simulink model "Exp4_19EE10011"  (R2021a)
settings: Solver=VariableStepAuto  StartTime=0.0  StopTime=3  RelTol=1e-3
libraries: spsSeriesRLCBranchLib x20, spsDiodeLib x13, spsCurrentMeasurementLib x11, spsVoltageMeasurementLib x9, spsThyristorLib x6, spsGroundLib x4, spsParallelRLCBranchLib x4, spsACVoltageSourceLib x3, spsLinearTransformerLib x3, spsRMSLib x2, spsMonostableLib x2, spsMosfetLib x2
settings Model: Creator=Asus  LastModifiedBy=Asus

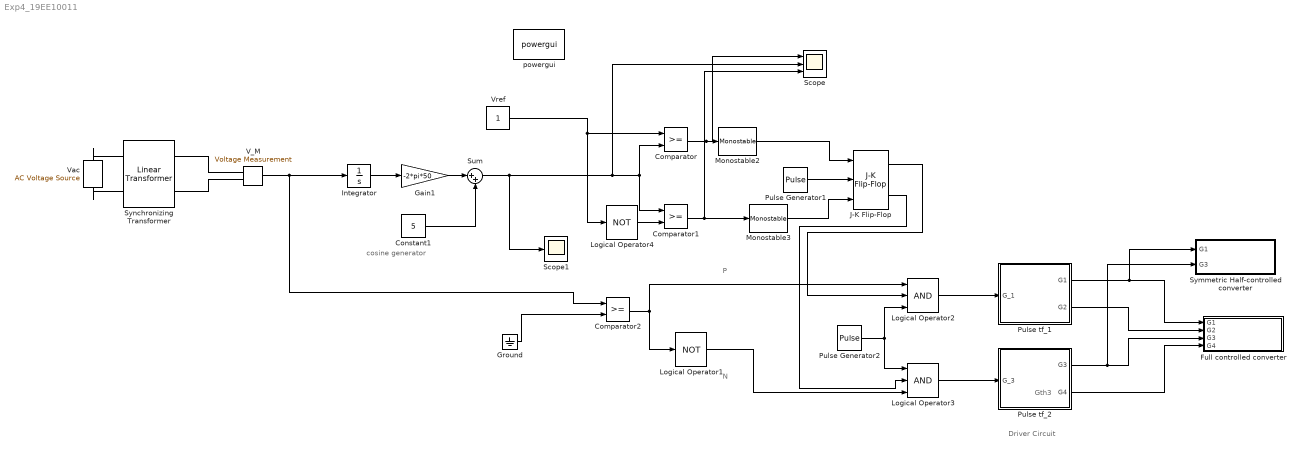
== system Exp4_19EE10011 ==
  note: Driver Circuit
  note: cosine generator
  note: P
  note: N
  note: Gth3
  Comparator : RelationalOperator  OutDataTypeStr=boolean  RndMeth=Nearest
  Comparator1 : RelationalOperator  OutDataTypeStr=boolean  RndMeth=Nearest
  Comparator2 : RelationalOperator  OutDataTypeStr=boolean  RndMeth=Nearest
  Constant1 : Constant  Value=5
  Full controlled converter : Subsystem
  Gain1 : Gain  Gain=-2*pi*50
  Ground : Ground
  Integrator : Integrator
  J-K Flip-Flop : simulink_extras/Flip Flops/J-K Flip-Flop  initial_condition=0
  Logical Operator1 : Logic  Operator=NOT  Inputs=inv  IconShape=distinctive  AllPortsSameDT=off  OutDataTypeStr=boolean
  Logical Operator2 : Logic  Inputs=3  IconShape=distinctive  AllPortsSameDT=off  OutDataTypeStr=boolean
  Logical Operator3 : Logic  Inputs=3  IconShape=distinctive  AllPortsSameDT=off  OutDataTypeStr=boolean
  Logical Operator4 : Logic  Operator=NOT  Inputs=inv  IconShape=distinctive  AllPortsSameDT=off  OutDataTypeStr=boolean
  Monostable2 : spsMonostableLib/Monostable  EdgeDetect=Rising  PulseDuration=10e-6  ic=0  Ts=0
      settings: SourceProductBaseCode=PS
  Monostable3 : spsMonostableLib/Monostable  EdgeDetect=Rising  PulseDuration=10e-6  ic=0  Ts=0
      settings: SourceProductBaseCode=PS
  Pulse Generator1 : DiscretePulseGenerator  PulseType=Time based  Period=2e-6  PulseWidth=50
  Pulse Generator2 : DiscretePulseGenerator  PulseType=Time based  Period=40e-6  PulseWidth=50
  Pulse tf_1 : Subsystem
  Pulse tf_2 : Subsystem
  Scope : Scope  NumInputPorts=3
  Scope1 : Scope
  Sum : Sum  Inputs=|++
  Symmetric Half-controlled converter : Subsystem
  Synchronizing Transformer : spsLinearTransformerLib/Linear Transformer  UNITS=SI  NominalPower=[ 4 50 ]  winding1="[230  6.90 7.1e-3]"  winding2=[3.605 0.0017 2.1e-6]  ThreeWindings=off  winding3=[3.15e+05 0.7938 0.084225]  RmLm=[600 1.145]  Measurements=None  DataType=on
  V_M : spsVoltageMeasurementLib/Voltage Measurement  PhasorSimulation=off  OutputType=Complex  PSBequivalent=0
  Vac : spsACVoltageSourceLib/AC Voltage Source  Amplitude=230  Phase=0  Frequency=50  SampleTime=0  Measurements=None  BusType=swing  Pref=10e3  Qref=0  Qmin=-inf  Qmax=+inf
  Vref : Constant
  powergui : spspowerguiLib/powergui  Priority=1  SimulationMode=Discrete  SampleTime=1e-6  frequency=60  Iterations=50  frequencyindice=50  Pbase=100e6  ErrMax=1e-4  UnitsV=kV  UnitsW=MW  buscounter=0  FunctionMessages=off  echomessages=off  EnableUseOfTLC=off  CurrentSourceSwitches=off  DisableSnubberDevices=off  DisableRonSwitches=off  DisableVfSwitches=off  DisplayEquations=off  AutomaticDiscreteSolvers=off  SolverType=Tustin/Backward Euler (TBE)  Interpol=off  ExternalGateDelay=off  methode=off  Ts=10  x0status=blocks  SPID=off  SwTol=0  HookPort=off  NonlinearTolerance=1e-4  nMaxIteration=100  ContinueOnMaxIteration=off  RestoreLinks=warning  ResistiveCurrentMeasurement=off  Frange=[0:2:500]  Ylog=off  Xlog=on  ShowGrid=off  save=off  variable=ZData  structure=ScopeData10  ZoomFFT=off  StartTime=0.124  cycles=2  DisplayStyle=2  fundamental=50  FreqAxis=on  MaxFrequency=5000  frequencyindicesteady=1  RmsSteady=1  display=off
  wires:
  Comparator/1 -> Scope/1, Monostable2/1
  J-K Flip-Flop/2 -> Logical Operator3/2
  Comparator1/1 -> Scope/3, Monostable3/1
  Monostable2/1 -> J-K Flip-Flop/1
  Logical Operator1/1 -> Logical Operator3/3
  Pulse Generator2/1 -> Logical Operator3/1, Logical Operator2/3
  Pulse Generator1/1 -> J-K Flip-Flop/2
  Ground/1 -> Comparator2/2
  Vref/1 -> Logical Operator4/1, Comparator/1
  J-K Flip-Flop/1 -> Logical Operator2/2
  Monostable3/1 -> J-K Flip-Flop/3
  Sum/1 -> Scope1/1, Comparator/2, Comparator1/1, Scope/2
  Comparator2/1 -> Logical Operator2/1, Logical Operator1/1
  Gain1/1 -> Sum/1
  Integrator/1 -> Gain1/1
  Constant1/1 -> Sum/2
  V_M/1 -> Integrator/1, Comparator2/1
  Logical Operator4/1 -> Comparator1/2
  Logical Operator2/1 -> Pulse tf_1/1(G_1)
  Logical Operator3/1 -> Pulse tf_2/1(G_3)
  Pulse tf_1/1(G1) -> Symmetric Half-controlled converter/1(G1), Full controlled converter/1(G1)
  Pulse tf_1/2(G2) -> Full controlled converter/2(G2)
  Pulse tf_2/1(G3) -> Symmetric Half-controlled converter/2(G3), Full controlled converter/3(G3)
  Pulse tf_2/2(G4) -> Full controlled converter/4(G4)
  connections:
  V_M/LConn2 -- Synchronizing Transformer/RConn2
  Vac/RConn1 -- Synchronizing Transformer/LConn1
  Vac/LConn1 -- Synchronizing Transformer/LConn2
  Synchronizing Transformer/RConn1 -- V_M/LConn1

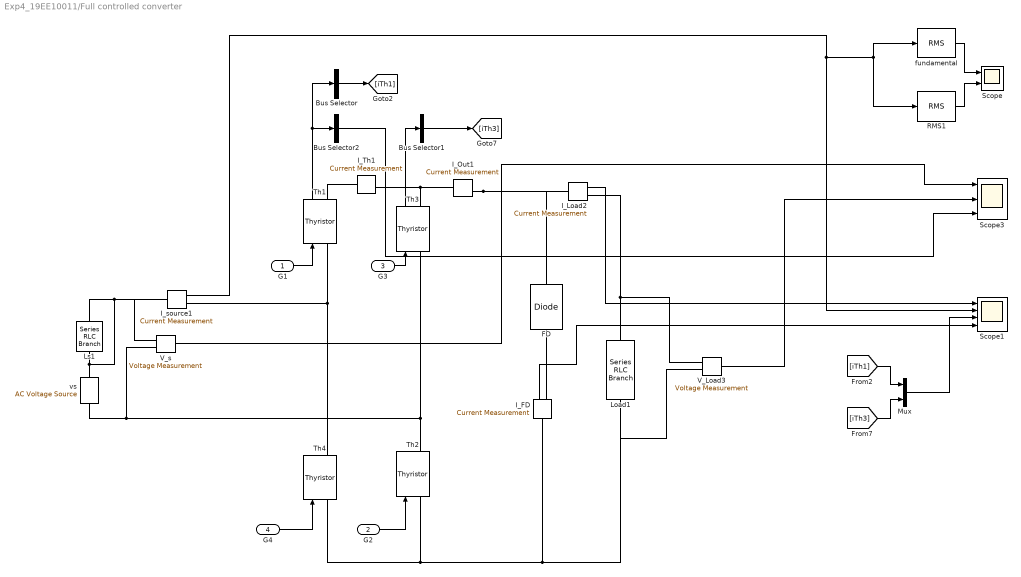
== system Exp4_19EE10011/Full controlled converter ==
  G1 : Inport
  G2 : Inport  Port=2
  G3 : Inport  Port=3
  G4 : Inport  Port=4
  Bus Selector : BusSelector  OutputSignals=Thyristor current  OutputAsBus=on
  Bus Selector1 : BusSelector  OutputSignals=Thyristor current  OutputAsBus=on
  Bus Selector2 : BusSelector  OutputSignals=Thyristor voltage  OutputAsBus=on
  FD : spsDiodeLib/Diode  Ron=0.14  Lon=0  Vf=0.6  IC=0  UseSnubber=off  Rs=500  Cs=250e-9  Measurements=off
  I_FD : spsCurrentMeasurementLib/Current Measurement  PhasorSimulation=off  OutputType=Complex  PSBequivalent=0
  I_Load2 : spsCurrentMeasurementLib/Current Measurement  PhasorSimulation=off  OutputType=Complex  PSBequivalent=0
  I_Out1 : spsCurrentMeasurementLib/Current Measurement  PhasorSimulation=off  OutputType=Complex  PSBequivalent=0
  I_Th1 : spsCurrentMeasurementLib/Current Measurement  PhasorSimulation=off  OutputType=Complex  PSBequivalent=0
  I_source1 : spsCurrentMeasurementLib/Current Measurement  PhasorSimulation=off  OutputType=Complex  PSBequivalent=0
  Load1 : spsSeriesRLCBranchLib/Series RLC Branch  LConnTagsString=__new0  RConnTagsString=__new0  BranchType=R  Resistance=22.4  Inductance=60e-3  SetiL0=off  InitialCurrent=0  Capacitance=1e-6  Setx0=off  InitialVoltage=0  Measurements=None
  Ls1 : spsSeriesRLCBranchLib/Series RLC Branch  LConnTagsString=__new0  RConnTagsString=__new0  BranchType=L  Resistance=0.01  Inductance=3.5e-3  SetiL0=off  InitialCurrent=0  Capacitance=1e-6  Setx0=off  InitialVoltage=0  Measurements=None
  Mux : Mux  Inputs=2
  RMS1 : spsRMSLib/RMS  TrueRMS=on  Freq=50  RMSInit=0  Ts=0
  Scope : Scope  NumInputPorts=2
  Scope1 : Scope  NumInputPorts=4
  Scope3 : Scope  NumInputPorts=3
  Th{1..4} (4 alike) : spsThyristorLib/Thyristor  Ron=0.05  Lon=0  Vf=1.5  IC=0  Rs=220  Cs=250e-9  Measurements=on
  V_Load3 : spsVoltageMeasurementLib/Voltage Measurement  PhasorSimulation=off  OutputType=Complex  PSBequivalent=0
  V_s : spsVoltageMeasurementLib/Voltage Measurement  PhasorSimulation=off  OutputType=Complex  PSBequivalent=0
  fundamental : spsRMSLib/RMS  TrueRMS=off  Freq=50  RMSInit=0  Ts=0
  vs : spsACVoltageSourceLib/AC Voltage Source  Amplitude=230  Phase=0  Frequency=50  SampleTime=0  Measurements=None  BusType=swing  Pref=10e3  Qref=0  Qmin=-inf  Qmax=+inf
  wires:
  Bus Selector/1 -> [iTh1]
  [iTh1] -> Mux/1
  I_FD/1 -> Scope1/4
  V_Load3/1 -> Scope3/2
  I_source1/1 -> Scope1/2, fundamental/1, RMS1/1
  G2/1 -> Th2/1
  Th1/1 -> Bus Selector/1, Bus Selector2/1
  G3/1 -> Th3/1
  G4/1 -> Th4/1
  Bus Selector2/1 -> Scope3/3
  RMS1/1 -> Scope/2
  Mux/1 -> Scope1/3
  G1/1 -> Th1/1
  I_Load2/1 -> Scope1/1
  V_s/1 -> Scope3/1
  Th3/1 -> Bus Selector1/1
  [iTh3] -> Mux/2
  Bus Selector1/1 -> [iTh3]
  fundamental/1 -> Scope/1
  connections:
  vs/LConn1 -- Th2/RConn1 -- Th3/LConn1 -- V_s/LConn2
  Th4/LConn1 -- I_FD/LConn1 -- Load1/RConn1 -- V_Load3/LConn2 -- Th2/LConn1
  I_Out1/LConn1 -- I_Th1/RConn1 -- Th3/RConn1
  V_Load3/LConn1 -- I_Load2/RConn1 -- Load1/LConn1
  Ls1/RConn1 -- Ls1/LConn1 -- V_s/LConn1 -- I_source1/LConn1 -- vs/RConn1
  I_source1/RConn1 -- Th4/RConn1 -- Th1/LConn1
  I_Out1/RConn1 -- FD/RConn1 -- I_Load2/LConn1
  Th1/RConn1 -- I_Th1/LConn1
  I_FD/RConn1 -- FD/LConn1

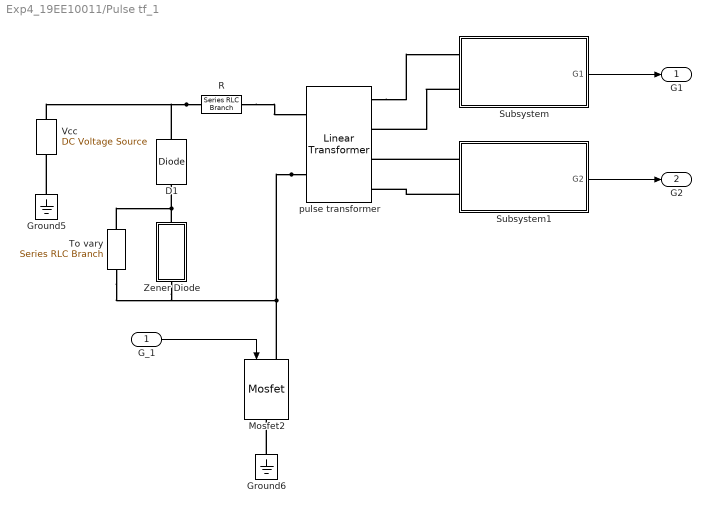
== system Exp4_19EE10011/Pulse tf_1 ==
  G_1 : Inport
  D1 : spsDiodeLib/Diode  Ron=0.001  Lon=0  Vf=0.7  IC=0  UseSnubber=off  Rs=inf  Cs=0  Measurements=off
  Ground5 : spsGroundLib/Ground  LConnTagsString=a
  Ground6 : spsGroundLib/Ground  LConnTagsString=a
  Mosfet2 : spsMosfetLib/Mosfet  Ron=0.1  Lon=0  Rd=0.01  Vfd=0  IC=0  Rs=1e5  Cs=inf  Measurements=off
  R : spsSeriesRLCBranchLib/Series RLC Branch  LConnTagsString=__new0  RConnTagsString=__new0  BranchType=R  Resistance=10  Inductance=60e-3  SetiL0=off  InitialCurrent=0  Capacitance=1e-6  Setx0=off  InitialVoltage=0  Measurements=None
  Subsystem : Subsystem
  Subsystem1 : Subsystem
  To vary : spsSeriesRLCBranchLib/Series RLC Branch  LConnTagsString=__new0  RConnTagsString=__new0  BranchType=R  Resistance=1e6  Inductance=60e-3  SetiL0=off  InitialCurrent=0  Capacitance=1e-6  Setx0=off  InitialVoltage=0  Measurements=None
  Vcc : spsDCVoltageSourceLib/DC Voltage Source  Amplitude=20  Measurements=None
  Zener Diode : Subsystem  mask(Zener Diode){Vz=30, Rzt=10, Rzk=400, Izm=10, Vf=0.7, Ron=1e-3}
      mask prompts: Vz "Zener Voltage Vz (V)"; Rzt "Dynamic Impedance Zzt (ohms)"; Rzk "Knee Impedance Zzk (ohms)"; Izm "Maximum Continuous Current Izm (A)"; Vf "Forward Voltage Drop Vf (V)"; Ron "On Resistance Ron (ohms)"
      mask help:
      | Implements a zener diode block.
      | Use values from standard datasheets to populate block dialog
  pulse transformer : spsLinearTransformerLib/Linear Transformer  UNITS=SI  NominalPower=[0.5 50e3 ]  winding1=[5 0.8 20e-6]  winding2=[5 0.8 20e-6]  ThreeWindings=on  winding3=[5 0.8 20e-6]  RmLm=[400 1.5e-3]  Measurements=None  DataType=on
  G1 : Outport
  G2 : Outport  Port=2
  wires:
  G_1/1 -> Mosfet2/1
  Subsystem1/1(G2) -> G2/1
  Subsystem/1(G1) -> G1/1
  connections:
  pulse transformer/LConn2 -- Mosfet2/LConn1 -- To vary/LConn1 -- Zener Diode/LConn1
  Ground6/LConn1 -- Mosfet2/RConn1
  Ground5/LConn1 -- Vcc/LConn1
  R/LConn1 -- pulse transformer/LConn1
  Zener Diode/RConn1 -- To vary/RConn1 -- D1/LConn1
  pulse transformer/RConn1 -- Subsystem/LConn1
  Subsystem/LConn2 -- pulse transformer/RConn2
  Subsystem1/LConn1 -- pulse transformer/RConn3
  Subsystem1/LConn2 -- pulse transformer/RConn4
  R/RConn1 -- D1/RConn1 -- Vcc/RConn1

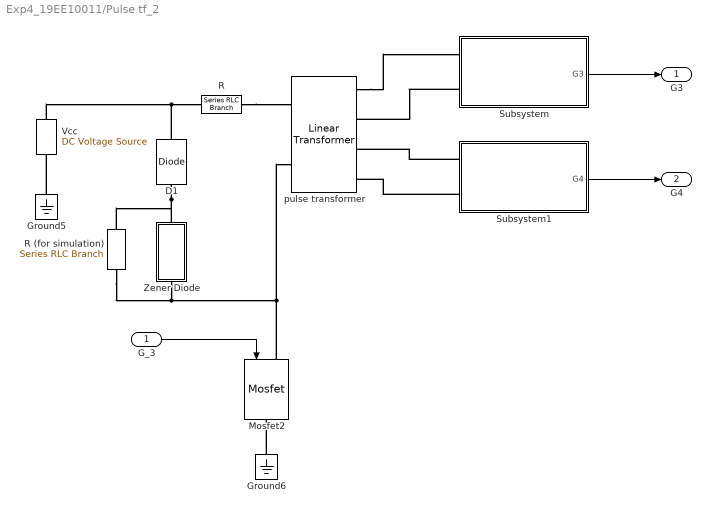
== system Exp4_19EE10011/Pulse tf_2 ==
  G_3 : Inport
  D1 : spsDiodeLib/Diode  Ron=0.001  Lon=0  Vf=0.7  IC=0  UseSnubber=off  Rs=inf  Cs=0  Measurements=off
  Ground5 : spsGroundLib/Ground  LConnTagsString=a
  Ground6 : spsGroundLib/Ground  LConnTagsString=a
  Mosfet2 : spsMosfetLib/Mosfet  Ron=0.1  Lon=0  Rd=0.01  Vfd=0  IC=0  Rs=1e5  Cs=inf  Measurements=off
  R : spsSeriesRLCBranchLib/Series RLC Branch  LConnTagsString=__new0  RConnTagsString=__new0  BranchType=R  Resistance=10  Inductance=60e-3  SetiL0=off  InitialCurrent=0  Capacitance=1e-6  Setx0=off  InitialVoltage=0  Measurements=None
  R (for simulation) : spsSeriesRLCBranchLib/Series RLC Branch  LConnTagsString=__new0  RConnTagsString=__new0  BranchType=R  Resistance=1e6  Inductance=60e-3  SetiL0=off  InitialCurrent=0  Capacitance=1e-6  Setx0=off  InitialVoltage=0  Measurements=None
  Subsystem : Subsystem
  Subsystem1 : Subsystem
  Vcc : spsDCVoltageSourceLib/DC Voltage Source  Amplitude=20  Measurements=None
  Zener Diode : Subsystem  mask(Zener Diode){Vz=30, Rzt=10, Rzk=400, Izm=10, Vf=0.7, Ron=1e-3}
      mask prompts: Vz "Zener Voltage Vz (V)"; Rzt "Dynamic Impedance Zzt (ohms)"; Rzk "Knee Impedance Zzk (ohms)"; Izm "Maximum Continuous Current Izm (A)"; Vf "Forward Voltage Drop Vf (V)"; Ron "On Resistance Ron (ohms)"
      mask help:
      | Implements a zener diode block.
      | Use values from standard datasheets to populate block dialog
  pulse transformer : spsLinearTransformerLib/Linear Transformer  UNITS=SI  NominalPower=[0.5 50e3 ]  winding1=[5 0.8 20e-6]  winding2=[5 0.8 20e-6]  ThreeWindings=on  winding3=[5 0.8 20e-6]  RmLm=[400 1.5e-3]  Measurements=None  DataType=on
  G3 : Outport
  G4 : Outport  Port=2
  wires:
  Subsystem/1(G3) -> G3/1
  Subsystem1/1(G4) -> G4/1
  G_3/1 -> Mosfet2/1
  connections:
  Vcc/RConn1 -- D1/RConn1 -- R/RConn1
  Subsystem1/LConn2 -- pulse transformer/RConn4
  Subsystem1/LConn1 -- pulse transformer/RConn3
  Subsystem/LConn2 -- pulse transformer/RConn2
  pulse transformer/RConn1 -- Subsystem/LConn1
  D1/LConn1 -- R (for simulation)/RConn1 -- Zener Diode/RConn1
  R/LConn1 -- pulse transformer/LConn1
  Ground5/LConn1 -- Vcc/LConn1
  Ground6/LConn1 -- Mosfet2/RConn1
  Zener Diode/LConn1 -- R (for simulation)/LConn1 -- Mosfet2/LConn1 -- pulse transformer/LConn2

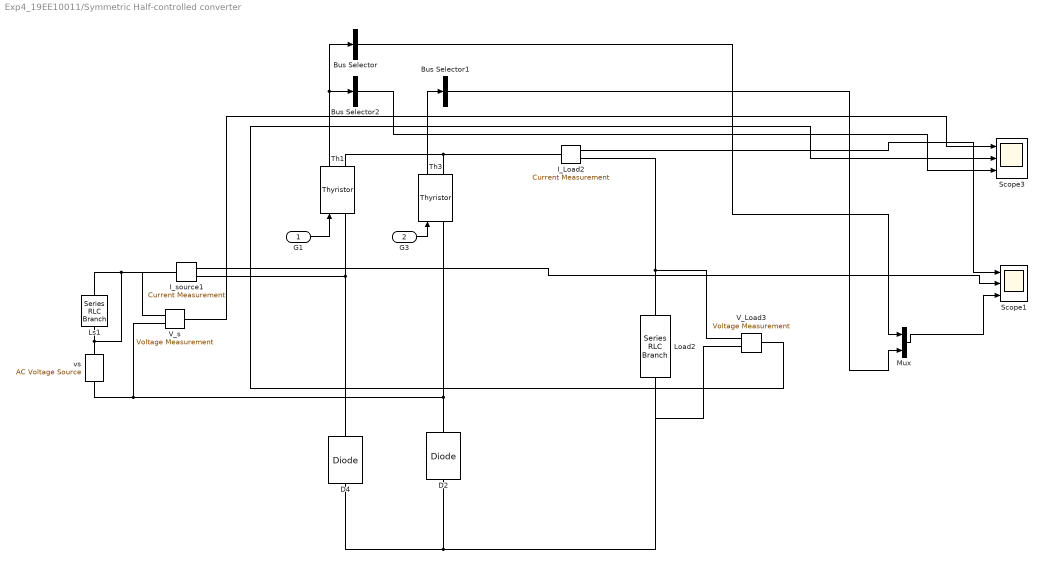
== system Exp4_19EE10011/Symmetric Half-controlled converter ==
  G1 : Inport
  G3 : Inport  Port=2
  Bus Selector : BusSelector  OutputSignals=Thyristor current  OutputAsBus=on
  Bus Selector1 : BusSelector  OutputSignals=Thyristor current  OutputAsBus=on
  Bus Selector2 : BusSelector  OutputSignals=Thyristor voltage  OutputAsBus=on
  D2 : spsDiodeLib/Diode  Ron=0.2  Lon=0  Vf=0.8  IC=0  UseSnubber=off  Rs=220  Cs=250e-9  Measurements=off
  D4 : spsDiodeLib/Diode  Ron=0.2  Lon=0  Vf=0.8  IC=0  UseSnubber=off  Rs=220  Cs=250e-9  Measurements=off
  I_Load2 : spsCurrentMeasurementLib/Current Measurement  PhasorSimulation=off  OutputType=Complex  PSBequivalent=0
  I_source1 : spsCurrentMeasurementLib/Current Measurement  PhasorSimulation=off  OutputType=Complex  PSBequivalent=0
  Load2 : spsSeriesRLCBranchLib/Series RLC Branch  LConnTagsString=__new0  RConnTagsString=__new0  BranchType=RL  Resistance=50  Inductance=60e-3  SetiL0=off  InitialCurrent=0  Capacitance=1e-6  Setx0=off  InitialVoltage=0  Measurements=None
  Ls1 : spsSeriesRLCBranchLib/Series RLC Branch  LConnTagsString=__new0  RConnTagsString=__new0  BranchType=L  Resistance=0.01  Inductance=3.5e-3  SetiL0=off  InitialCurrent=0  Capacitance=1e-6  Setx0=off  InitialVoltage=0  Measurements=None
  Mux : Mux  Inputs=2
  Scope1 : Scope  NumInputPorts=3
  Scope3 : Scope  NumInputPorts=3
  Th1 : spsThyristorLib/Thyristor  Ron=0.05  Lon=0  Vf=1.5  IC=0  Rs=220  Cs=250e-9  Measurements=on
  Th3 : spsThyristorLib/Thyristor  Ron=0.05  Lon=0  Vf=1.5  IC=0  Rs=220  Cs=250e-9  Measurements=on
  V_Load3 : spsVoltageMeasurementLib/Voltage Measurement  PhasorSimulation=off  OutputType=Complex  PSBequivalent=0
  V_s : spsVoltageMeasurementLib/Voltage Measurement  PhasorSimulation=off  OutputType=Complex  PSBequivalent=0
  vs : spsACVoltageSourceLib/AC Voltage Source  Amplitude=230  Phase=0  Frequency=50  SampleTime=0  Measurements=None  BusType=swing  Pref=10e3  Qref=0  Qmin=-inf  Qmax=+inf
  wires:
  G1/1 -> Th1/1
  Bus Selector2/1 -> Scope3/3
  Th3/1 -> Bus Selector1/1
  V_s/1 -> Scope3/1
  G3/1 -> Th3/1
  V_Load3/1 -> Scope3/2
  I_Load2/1 -> Scope1/1
  I_source1/1 -> Scope1/2
  Bus Selector/1 -> Mux/1
  Th1/1 -> Bus Selector/1, Bus Selector2/1
  Mux/1 -> Scope1/3
  Bus Selector1/1 -> Mux/2
  connections:
  D4/LConn1 -- D2/LConn1 -- V_Load3/LConn2 -- Load2/RConn1
  Ls1/RConn1 -- vs/RConn1 -- Ls1/LConn1 -- V_s/LConn1 -- I_source1/LConn1
  I_source1/RConn1 -- Th1/LConn1 -- D4/RConn1
  vs/LConn1 -- V_s/LConn2 -- Th3/LConn1 -- D2/RConn1
  I_Load2/LConn1 -- Th1/RConn1 -- Th3/RConn1
  Load2/LConn1 -- I_Load2/RConn1 -- V_Load3/LConn1

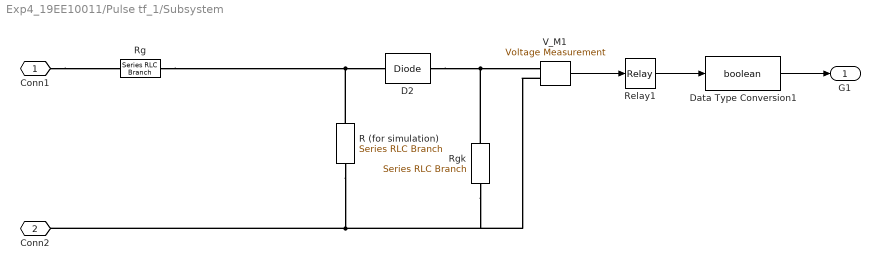
== system Exp4_19EE10011/Pulse tf_1/Subsystem ==
  D2 : spsDiodeLib/Diode  Ron=0.001  Lon=0  Vf=0.7  IC=0  UseSnubber=off  Rs=inf  Cs=0  Measurements=off
  Data Type Conversion1 : DataTypeConversion  OutDataTypeStr=boolean
  R (for simulation) : spsSeriesRLCBranchLib/Series RLC Branch  LConnTagsString=__new0  RConnTagsString=__new0  BranchType=R  Resistance=100000  Inductance=60e-3  SetiL0=off  InitialCurrent=0  Capacitance=1e-6  Setx0=off  InitialVoltage=0  Measurements=None
  Relay1 : Relay  OnSwitchValue=0.36  OffSwitchValue=0.1
  Rg : spsSeriesRLCBranchLib/Series RLC Branch  LConnTagsString=__new0  RConnTagsString=__new0  BranchType=R  Resistance=20  Inductance=60e-3  SetiL0=off  InitialCurrent=0  Capacitance=1e-6  Setx0=off  InitialVoltage=0  Measurements=None
  Rgk : spsSeriesRLCBranchLib/Series RLC Branch  LConnTagsString=__new0  RConnTagsString=__new0  BranchType=R  Resistance=10  Inductance=60e-3  SetiL0=off  InitialCurrent=0  Capacitance=1e-6  Setx0=off  InitialVoltage=0  Measurements=None
  V_M1 : spsVoltageMeasurementLib/Voltage Measurement  PhasorSimulation=off  OutputType=Complex  PSBequivalent=0
  Conn1 : PMIOPort  Side=Left
  Conn2 : PMIOPort  Port=2  Side=Left
  G1 : Outport
  wires:
  Data Type Conversion1/1 -> G1/1
  Relay1/1 -> Data Type Conversion1/1
  V_M1/1 -> Relay1/1
  connections:
  R (for simulation)/LConn1 -- Conn2/RConn1 -- V_M1/LConn2 -- Rgk/LConn1
  Conn1/RConn1 -- Rg/RConn1
  Rgk/RConn1 -- D2/RConn1 -- V_M1/LConn1
  R (for simulation)/RConn1 -- D2/LConn1 -- Rg/LConn1

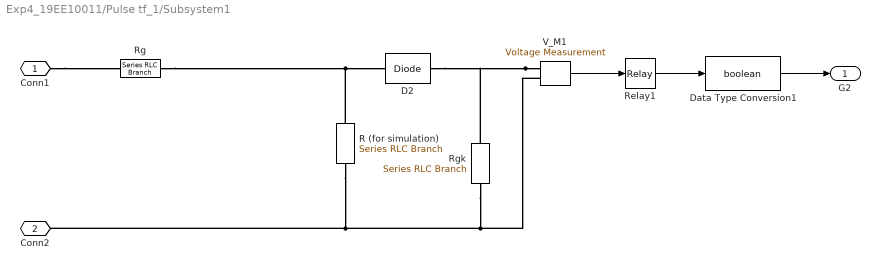
== system Exp4_19EE10011/Pulse tf_1/Subsystem1 ==
  D2 : spsDiodeLib/Diode  Ron=0.001  Lon=0  Vf=0.7  IC=0  UseSnubber=off  Rs=inf  Cs=0  Measurements=off
  Data Type Conversion1 : DataTypeConversion  OutDataTypeStr=boolean
  R (for simulation) : spsSeriesRLCBranchLib/Series RLC Branch  LConnTagsString=__new0  RConnTagsString=__new0  BranchType=R  Resistance=100000  Inductance=60e-3  SetiL0=off  InitialCurrent=0  Capacitance=1e-6  Setx0=off  InitialVoltage=0  Measurements=None
  Relay1 : Relay  OnSwitchValue=0.36  OffSwitchValue=0.1
  Rg : spsSeriesRLCBranchLib/Series RLC Branch  LConnTagsString=__new0  RConnTagsString=__new0  BranchType=R  Resistance=20  Inductance=60e-3  SetiL0=off  InitialCurrent=0  Capacitance=1e-6  Setx0=off  InitialVoltage=0  Measurements=None
  Rgk : spsSeriesRLCBranchLib/Series RLC Branch  LConnTagsString=__new0  RConnTagsString=__new0  BranchType=R  Resistance=10  Inductance=60e-3  SetiL0=off  InitialCurrent=0  Capacitance=1e-6  Setx0=off  InitialVoltage=0  Measurements=None
  V_M1 : spsVoltageMeasurementLib/Voltage Measurement  PhasorSimulation=off  OutputType=Complex  PSBequivalent=0
  Conn1 : PMIOPort  Side=Left
  Conn2 : PMIOPort  Port=2  Side=Left
  G2 : Outport
  wires:
  V_M1/1 -> Relay1/1
  Relay1/1 -> Data Type Conversion1/1
  Data Type Conversion1/1 -> G2/1
  connections:
  Rg/LConn1 -- D2/LConn1 -- R (for simulation)/RConn1
  V_M1/LConn1 -- D2/RConn1 -- Rgk/RConn1
  Conn1/RConn1 -- Rg/RConn1
  Rgk/LConn1 -- V_M1/LConn2 -- Conn2/RConn1 -- R (for simulation)/LConn1

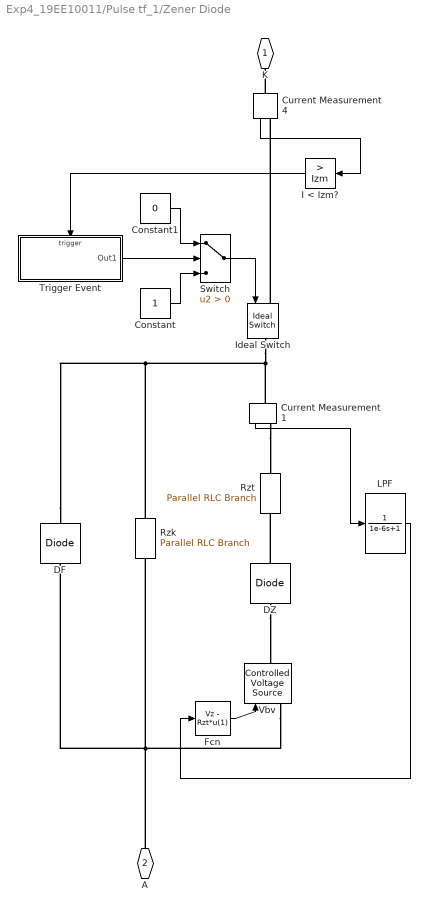
== system Exp4_19EE10011/Pulse tf_1/Zener Diode ==
  Constant : Constant
  Constant1 : Constant  Value=0
  Current Measurement1 : spsCurrentMeasurementLib/Current Measurement  PhasorSimulation=off  OutputType=Complex  PSBequivalent=0
  Current Measurement4 : spsCurrentMeasurementLib/Current Measurement  PhasorSimulation=off  OutputType=Complex  PSBequivalent=0
  DF : spsDiodeLib/Diode  Ron=Ron  Lon=0  Vf=Vf  IC=0  UseSnubber=off  Rs=1000  Cs=0  Measurements=off
      settings: AttributesFormatString=\n
  DZ : spsDiodeLib/Diode  Ron=1e-6  Lon=0  Vf=0  IC=0  UseSnubber=off  Rs=100  Cs=inf  Measurements=off
      settings: AttributesFormatString=\n
  Fcn : Fcn  Expr=Vz - Rzt*u(1)
  I < Izm? : simulink/Logic and Bit Operations/Compare To Constant  relop=>  const=Izm  OutDataTypeStr=boolean
  Ideal Switch : spsIdealSwitchLib/Ideal Switch  Ron=0.001  Lon=0  IC=1  Rs=1e5  Cs=0  Measurements=off
  LPF : TransferFcn  Denominator=[1e-6 1]
  Rzk : spsParallelRLCBranchLib/Parallel RLC Branch  LConnTagsString=a  RConnTagsString=__new0  BranchType=R  Resistance=Rzk  Inductance=1.0  SetiL0=off  InitialCurrent=0  Capacitance=1e-5  Setx0=off  InitialVoltage=0  Measurements=None
  Rzt : spsParallelRLCBranchLib/Parallel RLC Branch  LConnTagsString=a  RConnTagsString=__new0  BranchType=R  Resistance=Rzt  Inductance=1.0  SetiL0=off  InitialCurrent=0  Capacitance=1e-5  Setx0=off  InitialVoltage=0  Measurements=None
  Switch : Switch  Criteria=u2 > Threshold
  Trigger Event : Subsystem  TreatAsAtomicUnit=on
  Vbv : spsControlledVoltageSourceLib/Controlled Voltage Source  Initialize=off  Source_Type=DC  Amplitude=0  Phase=0  Frequency=0  Measurements=None
  K : PMIOPort  Side=Left
  A : PMIOPort  Port=2  Side=Right
  wires:
  Constant1/1 -> Switch/1
  Constant/1 -> Switch/3
  Trigger Event/1(Out1) -> Switch/2
  Switch/1 -> Ideal Switch/1
  I < Izm?/1 -> Trigger Event/Trigger
  LPF/1 -> Fcn/1
  Current Measurement1/1 -> LPF/1
  Current Measurement4/1 -> I < Izm?/1
  Fcn/1 -> Vbv/1
  connections:
  Vbv/LConn1 -- Rzk/LConn1 -- DF/LConn1 -- A/RConn1
  Ideal Switch/LConn1 -- Current Measurement4/RConn1
  DF/RConn1 -- Ideal Switch/RConn1 -- Current Measurement1/LConn1 -- Rzk/RConn1
  Current Measurement1/RConn1 -- Rzt/RConn1
  DZ/LConn1 -- Rzt/LConn1
  Current Measurement4/LConn1 -- K/RConn1
  DZ/RConn1 -- Vbv/RConn1

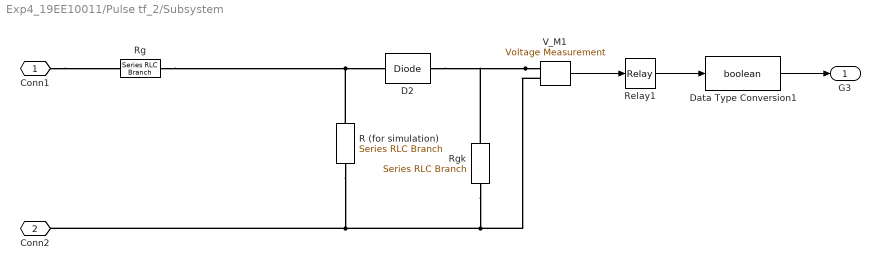
== system Exp4_19EE10011/Pulse tf_2/Subsystem ==
  D2 : spsDiodeLib/Diode  Ron=0.001  Lon=0  Vf=0.7  IC=0  UseSnubber=off  Rs=inf  Cs=0  Measurements=off
  Data Type Conversion1 : DataTypeConversion  OutDataTypeStr=boolean
  R (for simulation) : spsSeriesRLCBranchLib/Series RLC Branch  LConnTagsString=__new0  RConnTagsString=__new0  BranchType=R  Resistance=100000  Inductance=60e-3  SetiL0=off  InitialCurrent=0  Capacitance=1e-6  Setx0=off  InitialVoltage=0  Measurements=None
  Relay1 : Relay  OnSwitchValue=0.36  OffSwitchValue=0.1
  Rg : spsSeriesRLCBranchLib/Series RLC Branch  LConnTagsString=__new0  RConnTagsString=__new0  BranchType=R  Resistance=20  Inductance=60e-3  SetiL0=off  InitialCurrent=0  Capacitance=1e-6  Setx0=off  InitialVoltage=0  Measurements=None
  Rgk : spsSeriesRLCBranchLib/Series RLC Branch  LConnTagsString=__new0  RConnTagsString=__new0  BranchType=R  Resistance=10  Inductance=60e-3  SetiL0=off  InitialCurrent=0  Capacitance=1e-6  Setx0=off  InitialVoltage=0  Measurements=None
  V_M1 : spsVoltageMeasurementLib/Voltage Measurement  PhasorSimulation=off  OutputType=Complex  PSBequivalent=0
  Conn1 : PMIOPort  Side=Left
  Conn2 : PMIOPort  Port=2  Side=Left
  G3 : Outport
  wires:
  V_M1/1 -> Relay1/1
  Relay1/1 -> Data Type Conversion1/1
  Data Type Conversion1/1 -> G3/1
  connections:
  Rg/LConn1 -- D2/LConn1 -- R (for simulation)/RConn1
  V_M1/LConn1 -- D2/RConn1 -- Rgk/RConn1
  Conn1/RConn1 -- Rg/RConn1
  Rgk/LConn1 -- V_M1/LConn2 -- Conn2/RConn1 -- R (for simulation)/LConn1

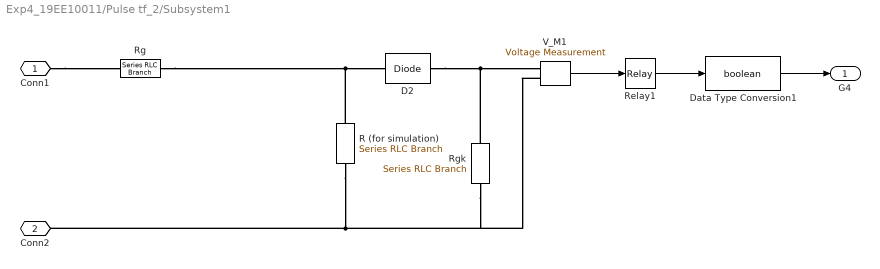
== system Exp4_19EE10011/Pulse tf_2/Subsystem1 ==
  D2 : spsDiodeLib/Diode  Ron=0.001  Lon=0  Vf=0.7  IC=0  UseSnubber=off  Rs=inf  Cs=0  Measurements=off
  Data Type Conversion1 : DataTypeConversion  OutDataTypeStr=boolean
  R (for simulation) : spsSeriesRLCBranchLib/Series RLC Branch  LConnTagsString=__new0  RConnTagsString=__new0  BranchType=R  Resistance=100000  Inductance=60e-3  SetiL0=off  InitialCurrent=0  Capacitance=1e-6  Setx0=off  InitialVoltage=0  Measurements=None
  Relay1 : Relay  OnSwitchValue=0.36  OffSwitchValue=0.1
  Rg : spsSeriesRLCBranchLib/Series RLC Branch  LConnTagsString=__new0  RConnTagsString=__new0  BranchType=R  Resistance=20  Inductance=60e-3  SetiL0=off  InitialCurrent=0  Capacitance=1e-6  Setx0=off  InitialVoltage=0  Measurements=None
  Rgk : spsSeriesRLCBranchLib/Series RLC Branch  LConnTagsString=__new0  RConnTagsString=__new0  BranchType=R  Resistance=10  Inductance=60e-3  SetiL0=off  InitialCurrent=0  Capacitance=1e-6  Setx0=off  InitialVoltage=0  Measurements=None
  V_M1 : spsVoltageMeasurementLib/Voltage Measurement  PhasorSimulation=off  OutputType=Complex  PSBequivalent=0
  Conn1 : PMIOPort  Side=Left
  Conn2 : PMIOPort  Port=2  Side=Left
  G4 : Outport
  wires:
  Data Type Conversion1/1 -> G4/1
  Relay1/1 -> Data Type Conversion1/1
  V_M1/1 -> Relay1/1
  connections:
  R (for simulation)/LConn1 -- Conn2/RConn1 -- V_M1/LConn2 -- Rgk/LConn1
  Conn1/RConn1 -- Rg/RConn1
  Rgk/RConn1 -- D2/RConn1 -- V_M1/LConn1
  R (for simulation)/RConn1 -- D2/LConn1 -- Rg/LConn1

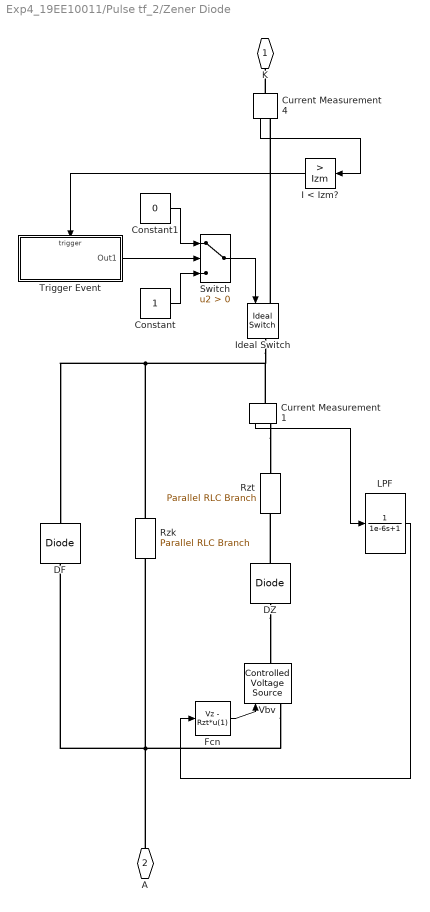
== system Exp4_19EE10011/Pulse tf_2/Zener Diode ==
  Constant : Constant
  Constant1 : Constant  Value=0
  Current Measurement1 : spsCurrentMeasurementLib/Current Measurement  PhasorSimulation=off  OutputType=Complex  PSBequivalent=0
  Current Measurement4 : spsCurrentMeasurementLib/Current Measurement  PhasorSimulation=off  OutputType=Complex  PSBequivalent=0
  DF : spsDiodeLib/Diode  Ron=Ron  Lon=0  Vf=Vf  IC=0  UseSnubber=off  Rs=1000  Cs=0  Measurements=off
      settings: AttributesFormatString=\n
  DZ : spsDiodeLib/Diode  Ron=1e-6  Lon=0  Vf=0  IC=0  UseSnubber=off  Rs=100  Cs=inf  Measurements=off
      settings: AttributesFormatString=\n
  Fcn : Fcn  Expr=Vz - Rzt*u(1)
  I < Izm? : simulink/Logic and Bit Operations/Compare To Constant  relop=>  const=Izm  OutDataTypeStr=boolean
  Ideal Switch : spsIdealSwitchLib/Ideal Switch  Ron=0.001  Lon=0  IC=1  Rs=1e5  Cs=0  Measurements=off
  LPF : TransferFcn  Denominator=[1e-6 1]
  Rzk : spsParallelRLCBranchLib/Parallel RLC Branch  LConnTagsString=a  RConnTagsString=__new0  BranchType=R  Resistance=Rzk  Inductance=1.0  SetiL0=off  InitialCurrent=0  Capacitance=1e-5  Setx0=off  InitialVoltage=0  Measurements=None
  Rzt : spsParallelRLCBranchLib/Parallel RLC Branch  LConnTagsString=a  RConnTagsString=__new0  BranchType=R  Resistance=Rzt  Inductance=1.0  SetiL0=off  InitialCurrent=0  Capacitance=1e-5  Setx0=off  InitialVoltage=0  Measurements=None
  Switch : Switch  Criteria=u2 > Threshold
  Trigger Event : Subsystem  TreatAsAtomicUnit=on
  Vbv : spsControlledVoltageSourceLib/Controlled Voltage Source  Initialize=off  Source_Type=DC  Amplitude=0  Phase=0  Frequency=0  Measurements=None
  K : PMIOPort  Side=Left
  A : PMIOPort  Port=2  Side=Right
  wires:
  Fcn/1 -> Vbv/1
  Current Measurement4/1 -> I < Izm?/1
  Current Measurement1/1 -> LPF/1
  LPF/1 -> Fcn/1
  I < Izm?/1 -> Trigger Event/Trigger
  Switch/1 -> Ideal Switch/1
  Trigger Event/1(Out1) -> Switch/2
  Constant/1 -> Switch/3
  Constant1/1 -> Switch/1
  connections:
  DZ/RConn1 -- Vbv/RConn1
  Current Measurement4/LConn1 -- K/RConn1
  DZ/LConn1 -- Rzt/LConn1
  Current Measurement1/RConn1 -- Rzt/RConn1
  Rzk/RConn1 -- Current Measurement1/LConn1 -- Ideal Switch/RConn1 -- DF/RConn1
  Ideal Switch/LConn1 -- Current Measurement4/RConn1
  A/RConn1 -- DF/LConn1 -- Rzk/LConn1 -- Vbv/LConn1

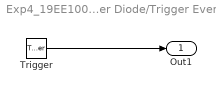
== system Exp4_19EE10011/Pulse tf_1/Zener Diode/Trigger Event ==
  Trigger : TriggerPort  VariantControl=Variant  ShowOutputPort=on
  Out1 : Outport
  wires:
  Trigger/1 -> Out1/1

== system Exp4_19EE10011/Pulse tf_2/Zener Diode/Trigger Event ==
  Trigger : TriggerPort  VariantControl=Variant  ShowOutputPort=on
  Out1 : Outport
  wires:
  Trigger/1 -> Out1/1
